simulink model "RoboBoat_AcousticTest_v2"  (R2014a)
settings: Solver=FixedStepDiscrete  StartTime=0.0  StopTime=inf  FixedStep=.1  RelTol=1e-3
undefined symbols (not defined in the file): Com1, Com2, Com3, Com4, DiscIntNeverNeededParam, standard
libraries: xpcseriallib x31, slrtlib x5, speedgoatlib_IO102 x5, speedgoatlib x1
(part 2 of 2)

== matlab function RoboBoat_AcousticTest_v2/Sensors/1020 Comms/MATLAB Function1 ==
  data: Valid input; Time input; asciiSEA output; Lat input; Long input; Color input; Depth input
% This function creates the underwater search message to be sent from 
% Speedgoat in ascii code
% Written by: Edward Zhu
% Date: 9/17/14

function asciiSEA = asciiSEAEncoder(Valid, Time, Lat, Long, Color, Depth)

% Initialize output message vector as the serial output block expects 128
% character message
asciiSEA = uint8(zeros(1,128));

% Convert static strings to ascii code
asciiMsgID = uint8('$RXSEA,');
asciiComma = uint8(',');
asciiDeciPt = uint8('.');
if Valid == 1
    if Lat >= 0
        asciiNS = uint8('N,');
    else
        Lat = -Lat;
        asciiNS = uint8('S,');
    end
    if Long >= 0
        asciiEW = uint8('E,');
    else
        Long = -Long;
        asciiEW = uint8('W,');
    end
else
    asciiNS = [32 asciiComma];
    asciiEW = [32 asciiComma];
end
asciiTeamID = uint8('FAUVU,');
asciiMsgEnd = uint8('*');
asciiMsgCRLF = [13 10];

% Convert UTC Time input (hhmmss) into ascii code
asciiTime = uint8(zeros(1,7));
asciiTime(7) = asciiComma;

for timeChar = 1:6
    asciiTime(timeChar) = floor(mod(Time,10^(7-timeChar))/...
        10^(6-timeChar)) + 48;
end

% Convert buoy color to ascii code (1 = R, 2 = G, 3 = B, 4 = W, 5 = K)
asciiColor = [uint8(32) asciiComma]; % Initialize as whitespace in case no buoy is found
if Valid == 1
    if Color == 1
        asciiColor(1) = uint8('R');
    elseif Color == 2
        asciiColor(1) = uint8('G');
    elseif Color == 3
        asciiColor(1) = uint8('B');
    elseif Color == 4
        asciiColor(1) = uint8('W');
    elseif Color == 5
        asciiColor(1) = uint8('K');
    end
end
% Convert latitude (dd.mmmmmm) into ascii code
asciiLat = uint8(zeros(1,10)+32); % Initialize as whitespace in case no buoy is found
asciiLat(10) = asciiComma;

% Only output values if valid bit is high
if Valid == 1
    asciiLat(3) = asciiDeciPt;
    latInt = floor(Lat);
    for latIntChar = 1:2
        asciiLat(latIntChar) = floor(mod(latInt,10^(3-latIntChar))/...
            10^(2-latIntChar)) + 48;
    end
    
    latDeci = mod(Lat,latInt) * 10^6;
    for latDeciChar = 1:6
        asciiLat(latDeciChar+3) = floor(mod(latDeci,10^(7-latDeciChar))/...
            10^(6-latDeciChar)) + 48;
    end
end

% Convert longitude (ddd.mmmmmm) into ascii code
asciiLong = uint8(zeros(1,11)+32); % Initialize as whitespace in case no buoy is found
asciiLong(11) = asciiComma;

% Only output values if valid bit is high
if Valid == 1
    asciiLong(4) = asciiDeciPt;
    longInt = floor(Long);
    for longIntChar = 1:3
        asciiLong(longIntChar) = floor(mod(longInt,10^(4-longIntChar))/...
            10^(3-longIntChar)) + 48;
    end
    
    longDeci = mod(Long,longInt) * 10^6;
    for longDeciChar = 1:6
        asciiLong(longDeciChar+4) = floor(mod(longDeci,10^(7-longDeciChar))/...
            10^(6-longDeciChar)) + 48;
    end
end

% Convert depth (m) (##.##) into ascii
asciiDepth = uint8(zeros(1,6)+32); % Initialize as whitespace in case no buoy is found
asciiDepth(6) = asciiMsgEnd;

% Only output values if valid bit is high
if Valid == 1
    asciiDepth(3) = asciiDeciPt;
    depthInt = floor(Depth);
    for depthIntChar = 1:2
        asciiDepth(depthIntChar) = floor(mod(depthInt,10^(3-depthIntChar))/...
            10^(2-depthIntChar)) + 48;
    end
    
    depthDeci = mod(Depth,depthInt) * 10^2;
    for depthDeciChar = 1:2
        asciiDepth(depthDeciChar+3) = floor(mod(depthDeci,10^(3-depthDeciChar))/...
            10^(2-depthDeciChar)) + 48;
    end
end

% Concat individual ascii arrays into one array
asciiPreChkSum = cat(2,asciiMsgID,asciiTime,asciiTeamID,asciiColor,...
    asciiLat,asciiNS,asciiLong,asciiEW,asciiDepth);

% Calculate the checksum of the message from the '$' to the '*' and convert
% to hex
chkSum = uint8(0);

for chksumChar = 1:(length(asciiPreChkSum)-2)
    chkSum = bitxor(chkSum,asciiPreChkSum(chksumChar+1));
end

% Convert the checksum to ascii
chkSum = dec2hex(chkSum);
asciiChkSum = uint8(zeros(1,length(chkSum))+32);
for i = 1:length(chkSum)
    asciiChkSum(i) = uint8(chkSum(i));
end

% Concat the checksum and the '/r/n' to the end of the message
asciiPostChkSum = cat(2,asciiPreChkSum,asciiChkSum,asciiMsgCRLF);

% Output the final message
asciiSEA(1:length(asciiPostChkSum)) = asciiPostChkSum;

== matlab function RoboBoat_AcousticTest_v2/Sensors/1020 Comms/MATLAB Function2 ==
  data: Time input; asciiLIT output; Sequence input
% This function creates the light tower message to be sent from 
% Speedgoat in ascii code
% Written by: Edward Zhu
% Date: 9/17/14

function asciiLIT = asciiLITEncoder(Time, Sequence)

% Initialize output message vector as the serial output block expects 128
% character message
asciiLIT = uint8(zeros(1,128));

% Convert static strings to ascii code
asciiMsgID = uint8('$RXLIT,');
asciiComma = uint8(',');
asciiTeamID = uint8('FAUVU,');
asciiMsgEnd = uint8('*');
asciiMsgCRLF = [13 10];

% Convert UTC Time input (hhmmss) into ascii code
asciiTime = uint8(zeros(1,7));
asciiTime(7) = asciiComma;

for timeChar = 1:6
    asciiTime(timeChar) = floor(mod(Time,10^(7-timeChar))/...
        10^(6-timeChar)) + 48;
end

% Convert the light sequece into ascii code (1 = R, 2 = B, 3 = G)
asciiSeq = uint8(zeros(1,4)+32);
asciiSeq(4) = asciiMsgEnd;

if Sequence(1) > 0 && Sequence(2) > 0 && Sequence(3) > 0
    for seqChar = 1:3
        if Sequence(seqChar) == 1
            Sequence(seqChar) = uint8('R');
        elseif Sequence(seqChar) == 2
            Sequence(seqChar) = uint8('B');
        elseif Sequence(seqChar) == 3
            Sequence(seqChar) = uint8('G');
        end
    end
    asciiSeq(1:3) = Sequence;
end

% Concat individual ascii arrays into one array
asciiPreChkSum = cat(2,asciiMsgID,asciiTime,asciiTeamID,asciiSeq);

% Calculate the checksum of the message from the '$' to the '*' and convert
% to hex
chkSum = uint8(0);

for chksumChar = 1:(length(asciiPreChkSum)-2)
    chkSum = bitxor(chkSum,asciiPreChkSum(chksumChar+1));
end

% Convert the checksum to ascii
chkSum = dec2hex(chkSum);
asciiChkSum = uint8(zeros(1,length(chkSum))+32);
for i = 1:length(chkSum)
    asciiChkSum(i) = uint8(chkSum(i));
end

% Concat the checksum and the '/r/n' to the end of the message
asciiPostChkSum = cat(2,asciiPreChkSum,asciiChkSum,asciiMsgCRLF);

% Output the final message
asciiLIT(1:length(asciiPostChkSum)) = asciiPostChkSum;

== matlab function RoboBoat_AcousticTest_v2/Sensors/1020 Comms/MATLAB Function3 ==
  data: Time input; asciiHRT output; Lat input; Long input; Mode input; Task input
% This function creates the heartbeat message to be sent from Speedgoat in
% ascii code
% Written by: Edward Zhu
% Date: 9/17/14

function asciiHRT = asciiHRTEncoder(Time, Lat, Long, Mode, Task)

% Initialize output message vector as the serial output block expects 128
% character message
asciiHRT = uint8(zeros(1,128));

% Convert static strings to ascii code
asciiMsgID = uint8('$RXHRT,');
asciiComma = uint8(',');
asciiDeciPt = uint8('.');
if Lat >= 0
    asciiNS = uint8('N,');
else
    Lat = -Lat;
    asciiNS = uint8('S,');
end
if Long >= 0
    asciiEW = uint8('E,');
else
    Long = -Long;
    asciiEW = uint8('W,');
end
asciiTeamID = uint8('FAUVU,');
asciiMsgEnd = uint8('*');
asciiMsgCRLF = [13 10];

% Convert UTC Time input (hhmmss) into ascii code
asciiTime = uint8(zeros(1,7));
asciiTime(7) = asciiComma;

for timeChar = 1:6
    asciiTime(timeChar) = floor(mod(Time,10^(7-timeChar))/...
        10^(6-timeChar)) + 48;
end

% Convert latitude (dd.mmmmmm) into ascii code
asciiLat = uint8(zeros(1,10));
asciiLat(10) = asciiComma;
asciiLat(3) = asciiDeciPt;

latInt = floor(Lat);
for latIntChar = 1:2
    asciiLat(latIntChar) = floor(mod(latInt,10^(3-latIntChar))/...
        10^(2-latIntChar)) + 48;
end

latDeci = mod(Lat,latInt) * 10^6;
for latDeciChar = 1:6
    asciiLat(latDeciChar+3) = floor(mod(latDeci,10^(7-latDeciChar))/...
        10^(6-latDeciChar)) + 48;
end

% Convert longitude (ddd.mmmmmm) into ascii code
asciiLong = uint8(zeros(1,11));
asciiLong(11) = asciiComma;
asciiLong(4) = asciiDeciPt;

longInt = floor(Long);
for longIntChar = 1:3
    asciiLong(longIntChar) = floor(mod(longInt,10^(4-longIntChar))/...
        10^(3-longIntChar)) + 48;
end

longDeci = mod(Long,longInt) * 10^6;
for longDeciChar = 1:6
    asciiLong(longDeciChar+4) = floor(mod(longDeci,10^(7-longDeciChar))/...
        10^(6-longDeciChar)) + 48;
end

% Convert vehicle mode into ascii (1 = RC, 2 = Auto)
if Mode ~= 1 || Mode ~= 2
    Mode = 1;
    asciiMode = [uint8(Mode+48) asciiComma];
else
    asciiMode = [uint8(Mode+48) asciiComma];
end

% Convert vehicle task into ascii
asciiTask = [uint8(Task+48) asciiMsgEnd];

% Concat individual ascii arrays into one array
asciiPreChkSum = cat(2,asciiMsgID,asciiTime,asciiLat,asciiNS,asciiLong,asciiEW,...
    asciiTeamID,asciiMode,asciiTask);

% Calculate the checksum of the message from the '$' to the '*' and convert
% to hex
chkSum = uint8(0);

for chksumChar = 1:(length(asciiPreChkSum)-2)
    chkSum = bitxor(chkSum,asciiPreChkSum(chksumChar+1));
end

% Convert the checksum to ascii
chkSum = dec2hex(chkSum);
asciiChkSum = uint8(zeros(1,length(chkSum))+32);
for i = 1:length(chkSum)
    asciiChkSum(i) = uint8(chkSum(i));
end

% Concat the checksum and the '/r/n' to the end of the message
asciiPostChkSum = cat(2,asciiPreChkSum,asciiChkSum,asciiMsgCRLF);

% Output the final message
asciiHRT(1:length(asciiPostChkSum)) = asciiPostChkSum;
